simulink model "Stewart_NMPC"  (R2017b)
settings: Solver=VariableStepAuto  StartTime=0.0  StopTime=T  RelTol=1e-3  EnableMultiTasking=on
values from neighbouring files (symbols this model uses):
  c = corrcoef(y(i,:)', r(i,:)')    [main.m]
  x0 = MPC.Xlb + rand(12,1).*(MPC.Xub - MPC.Xlb)    [Regressioin_Approximate_NMPC.m]    (also in find_optimal_NMPC.m = [0,0,0,0,0,0])
settings Model: Creator=Administrator  LastModifiedBy=Administrator
settings DataIOCC: LimitDataPoints=on
settings OptimizationCC: LifeSpan=inf
settings DebuggingCC: AllowSymbolicDim=off  SFUnexpectedBacktrackingDiag=warning  SFNoUnconditionalDefaultTransitionDiag=warning  SFExecutionAtInitializationDiag=none
settings CodeAppCC: StateflowObjectComments=on
settings GRTTargetCC: TargetLangStandard=C89/C90 (ANSI)  GeneratePreprocessorConditionals=Disable all
settings ConfigComp: CovMetricSettings=dw  CovHtmlReporting=on  CovSaveCumulativeToWorkspaceVar=on  CovSaveSingleToWorkspaceVar=on  CovExternalEMLEnable=off  CovSFcnEnable=off
settings SimscapeCC: SimscapeNominalValues="[{\"value\":\"10\",\"unit\":\"V\"},{\"value\":\"1\",\"unit\":\"A\"},{\"value\":\"10\",\"unit\":\"N*m\"},{\"value\":\"10\",\"unit\":\"bar\"},{\"value\":\"100\",\"unit\":\"kJ/kg\"},{\"value\":\"1\",\"unit\":\"kW\"},{\"value\":\"300\",\"unit\":\"K\"},{\"value\":\"100\",\"unit\":\"cm^3/s\"},{\"value\":\"1\",\"unit\":\"kN\"},{\"value\":\"1\",\"unit\":\"g/cm^3\"},{\"value\":\"1\",\"unit\":\"l\"},{\"value\":\"1\",\"unit\":\"cm^2\"},{\"value\":\"60\",\"unit\":\"Hz\"}]"  SimscapeLogType=all  SimscapeLogDataHistory=10000
settings ConfigurationSet: Description=SimMechanics 2G

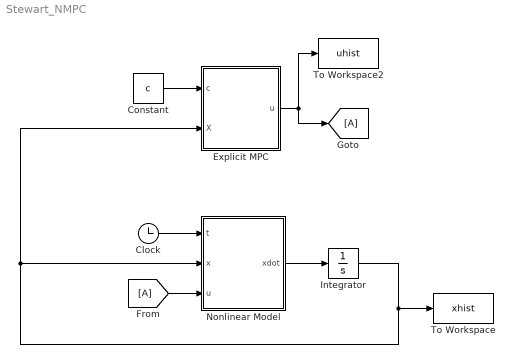
== system Stewart_NMPC ==
  Clock : Clock
  Constant : Constant  Value=c
  Explicit MPC : MATLAB Function  TreatAsAtomicUnit=on
  Integrator : Integrator  InitialCondition=x0
  Nonlinear Model : MATLAB Function  TreatAsAtomicUnit=on
  To Workspace : ToWorkspace  VariableName=xhist  SaveFormat=Timeseries  SampleTime=-1
  To Workspace2 : ToWorkspace  VariableName=uhist  SaveFormat=Timeseries  SampleTime=-1
  wires:
  Explicit MPC/1(u) -> [A], To Workspace2/1
  Clock/1 -> Nonlinear Model/1(t)
  [A] -> Nonlinear Model/3(u)
  Integrator/1 -> To Workspace/1, Explicit MPC/2(X), Nonlinear Model/2(x)
  Nonlinear Model/1(xdot) -> Integrator/1
  Constant/1 -> Explicit MPC/1(c)

== matlab function Stewart_NMPC/Nonlinear Model ==
  data: xdot output; t input; x input; u input
function xdot = fcn(t, x, u)

xdot = [x(2) + u*(0.5 + 0.5*x(1));...
     x(1) + u*(0.5 - 2.0*x(2))];

== matlab function Stewart_NMPC/Explicit MPC ==
  data: u output; c input; X input
function u = fcn(c, X)

% Basis functions
S = @(x,y) [1, x, y, x*y, (2*x^2-1)*y, (2*y^2-1)*x,...
            (4*x^3 - 3*x), (4*y^3 - 3*y)];

% Computing approx NMPC
u = S(X(1), X(2))*c;

% Projection
if u > 2
    u = 2;
end

if u < -2
    u = -2;
end
